simulink model "MasterSubsystems"  (R2021b)
settings: Solver=FixedStepDiscrete  StartTime=0.0  StopTime=10.0  FixedStep=0.001  RelTol=1e-3
undefined symbols (not defined in the file): DiscIntNeverNeededParam
libraries: slpidlib x2
settings Model: TunableVars=dt,k1  TunableVarsStorageClass=Auto,Auto  TunableVarsTypeQualifier=,  Creator=rrai-HIL  LastModifiedBy=rrai-HIL
settings ConfigComp: PLC_TargetIDE=plcopen  PLC_MultiTBSigbuilderTimeRange=off  PLC_ReuseMLFcnVariable=on  PLC_InlineEnumCastFunction=off

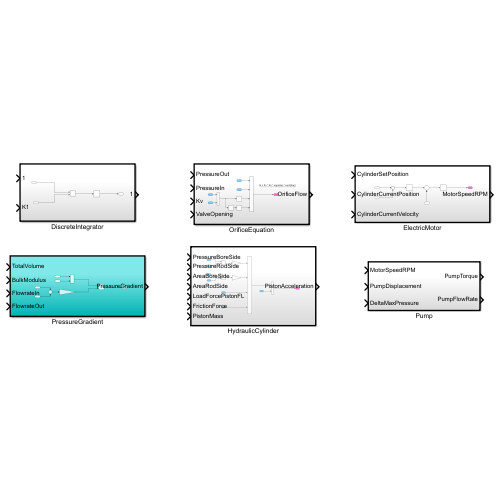
[thumbnail: Simulink's stored preview of the top-level diagram]
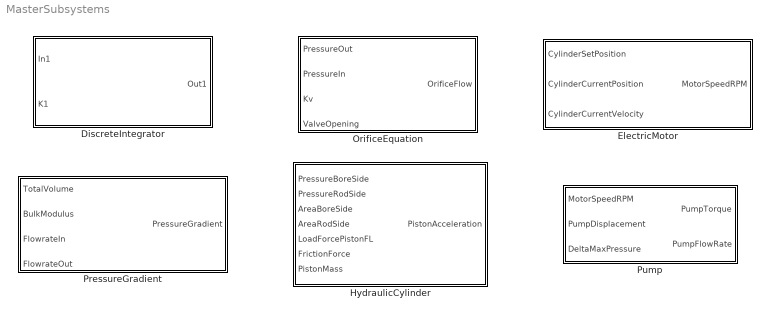
== system MasterSubsystems ==
  DiscreteIntegrator : Subsystem  TreatAsAtomicUnit=on
  ElectricMotor : Subsystem  TreatAsAtomicUnit=on
  HydraulicCylinder : Subsystem  TreatAsAtomicUnit=on
  OrificeEquation : Subsystem  TreatAsAtomicUnit=on
  PressureGradient : Subsystem  TreatAsAtomicUnit=on
  Pump : Subsystem  TreatAsAtomicUnit=on

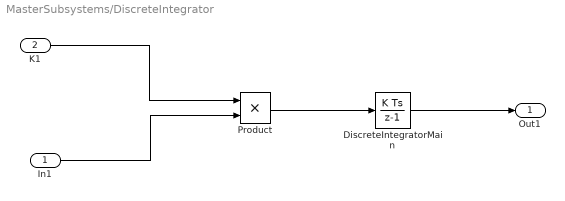
== system MasterSubsystems/DiscreteIntegrator ==
  In1 : Inport  OutDataTypeStr=single
  K1 : Inport  Port=2  OutDataTypeStr=single
  DiscreteIntegratorMain : DiscreteIntegrator  SampleTime=-1  ICPrevOutput=DiscIntNeverNeededParam  ICPrevScaledInput=DiscIntNeverNeededParam
  Product : Product
  Out1 : Outport  OutDataTypeStr=single
  wires:
  DiscreteIntegratorMain/1 -> Out1/1
  In1/1 -> Product/2
  Product/1 -> DiscreteIntegratorMain/1
  K1/1 -> Product/1

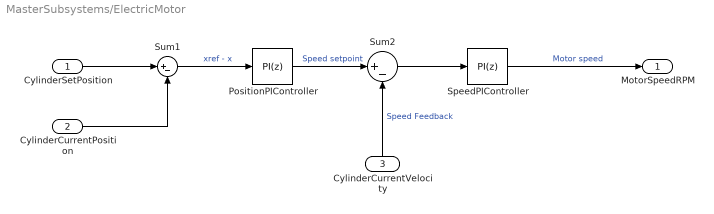
== system MasterSubsystems/ElectricMotor ==
  CylinderSetPosition : Inport
  CylinderCurrentPosition : Inport  Port=2
  CylinderCurrentVelocity : Inport  Port=3
  PositionPIController : slpidlib/PID Controller  Controller=PI  Form=Parallel  TimeDomain=Discrete-time  UseExternalTs=off  SampleTime=-1  IntegratorMethod=Forward Euler  FilterMethod=Forward Euler  ControllerParametersSource=internal  P=5  I=0.001  D=0  UseFilter=on  N=100  TunerSelectOption=Transfer Function Based (PID Tuner App)  InitialConditionSource=internal  InitialConditionForIntegrator=0  InitialConditionForFilter=0  DifferentiatorICPrevScaledInput=0  ExternalReset=none  TrackingMode=off  Kt=1  LimitOutput=on  SatLimitsSource=internal  UpperSaturationLimit=0.23  LowerSaturationLimit=-0.23  LinearizeAsGain=on  AntiWindupMode=none  Kb=1  POutMin=[]  POutMax=[]  IOutMin=[]  IOutMax=[]  DOutMin=[]  DOutMax=[]  NOutMin=[]  NOutMax=[]  SumOutMin=[]  SumOutMax=[]  SaturationOutMin=[]  SaturationOutMax=[]  PParamMin=[]  PParamMax=[]  IParamMin=[]  IParamMax=[]  DParamMin=[]  DParamMax=[]  NParamMin=[]  NParamMax=[]  KbParamMin=[]  KbParamMax=[]  KtParamMin=[]  KtParamMax=[]  KbOutMin=[]  KbOutMax=[]  KtOutMin=[]  KtOutMax=[]  IntegratorOutMin=[]  IntegratorOutMax=[]  FilterOutMin=[]  FilterOutMax=[]  SumI1OutMin=[]  SumI1OutMax=[]  SumI2OutMin=[]  SumI2OutMax=[]  SumI3OutMin=[]  SumI3OutMax=[]  SumI4OutMin=[]  SumI4OutMax=[]  SumDOutMin=[]  SumDOutMax=[]  DifferentiatorOutMin=[]  DifferentiatorOutMax=[]  FilterDiffOutCoefMin=[]  FilterDiffOutCoefMax=[]  ReciprocalOutMin=[]  ReciprocalOutMax=[]  SumDenOutMin=[]  SumDenOutMax=[]  SumNumOutMin=[]  SumNumOutMax=[]  DivideOutMin=[]  DivideOutMax=[]  UdiffTsProdOutMin=[]  UdiffTsProdOutMax=[]  NTsProdOutMin=[]  NTsProdOutMax=[]  UintegralTsProdOutMin=[]  UintegralTsProdOutMax=[]  UngainTsProdOutMin=[]  UngainTsProdOutMax=[]  IntegratorContinuousStateAttributes=''  IntegratorStateMustResolveToSignalObject=off  IntegratorRTWStateStorageClass=Auto  FilterContinuousStateAttributes=''  FilterStateMustResolveToSignalObject=off  FilterRTWStateStorageClass=Auto  ParallelPVariant=InternalParameters  IdealPVariant=Disabled  IVariant=InternalParameters  DVariant=Disabled  IntegratorVariant=Discrete  SatVariant=Enabled  AWVariant=Passthrough  PCopyVariant=Disabled  TRVariant=Disabled  FdbkBlocksVariant=Forward  IdealPFdbkVariant=Disabled  SatFdbkVariant=Disabled  DerivativeFilterVariant=Disabled  NVariant=Disabled  NCopyVariant=Disabled_SignalSpec  FilterICVariant=Disabled  IntegratorICVariant=InternalICs  ExternalResetVariant=Disabled  TRSumVariant=Passthrough  SumFdbkVariant=Disabled  SumVariant=Sum_PI  TsampFilterVariant=InternalTs  TsampNgainVariant=Passthrough  TsampIntegralVariant=Passthrough  ExternalSaturationOutDataTypeStr=Inherit: Same as second input
  SpeedPIController : slpidlib/PID Controller  Controller=PI  Form=Parallel  TimeDomain=Discrete-time  UseExternalTs=off  SampleTime=-1  IntegratorMethod=Forward Euler  FilterMethod=Forward Euler  ControllerParametersSource=internal  P=2000  I=0.01  D=0  UseFilter=on  N=100  TunerSelectOption=Transfer Function Based (PID Tuner App)  InitialConditionSource=internal  InitialConditionForIntegrator=0  InitialConditionForFilter=0  DifferentiatorICPrevScaledInput=0  ExternalReset=none  TrackingMode=off  Kt=1  LimitOutput=off  SatLimitsSource=internal  UpperSaturationLimit=0.23  LowerSaturationLimit=-0.23  LinearizeAsGain=on  AntiWindupMode=none  Kb=1  POutMin=[]  POutMax=[]  IOutMin=[]  IOutMax=[]  DOutMin=[]  DOutMax=[]  NOutMin=[]  NOutMax=[]  SumOutMin=[]  SumOutMax=[]  SaturationOutMin=[]  SaturationOutMax=[]  PParamMin=[]  PParamMax=[]  IParamMin=[]  IParamMax=[]  DParamMin=[]  DParamMax=[]  NParamMin=[]  NParamMax=[]  KbParamMin=[]  KbParamMax=[]  KtParamMin=[]  KtParamMax=[]  KbOutMin=[]  KbOutMax=[]  KtOutMin=[]  KtOutMax=[]  IntegratorOutMin=[]  IntegratorOutMax=[]  FilterOutMin=[]  FilterOutMax=[]  SumI1OutMin=[]  SumI1OutMax=[]  SumI2OutMin=[]  SumI2OutMax=[]  SumI3OutMin=[]  SumI3OutMax=[]  SumI4OutMin=[]  SumI4OutMax=[]  SumDOutMin=[]  SumDOutMax=[]  DifferentiatorOutMin=[]  DifferentiatorOutMax=[]  FilterDiffOutCoefMin=[]  FilterDiffOutCoefMax=[]  ReciprocalOutMin=[]  ReciprocalOutMax=[]  SumDenOutMin=[]  SumDenOutMax=[]  SumNumOutMin=[]  SumNumOutMax=[]  DivideOutMin=[]  DivideOutMax=[]  UdiffTsProdOutMin=[]  UdiffTsProdOutMax=[]  NTsProdOutMin=[]  NTsProdOutMax=[]  UintegralTsProdOutMin=[]  UintegralTsProdOutMax=[]  UngainTsProdOutMin=[]  UngainTsProdOutMax=[]  IntegratorContinuousStateAttributes=''  IntegratorStateMustResolveToSignalObject=off  IntegratorRTWStateStorageClass=Auto  FilterContinuousStateAttributes=''  FilterStateMustResolveToSignalObject=off  FilterRTWStateStorageClass=Auto  ParallelPVariant=InternalParameters  IdealPVariant=Disabled  IVariant=InternalParameters  DVariant=Disabled  IntegratorVariant=Discrete  SatVariant=Disabled  AWVariant=Passthrough  PCopyVariant=Disabled  TRVariant=Disabled  FdbkBlocksVariant=Forward  IdealPFdbkVariant=Disabled  SatFdbkVariant=Disabled  DerivativeFilterVariant=Disabled  NVariant=Disabled  NCopyVariant=Disabled_SignalSpec  FilterICVariant=Disabled  IntegratorICVariant=InternalICs  ExternalResetVariant=Disabled  TRSumVariant=Passthrough  SumFdbkVariant=Disabled  SumVariant=Sum_PI  TsampFilterVariant=InternalTs  TsampNgainVariant=Passthrough  TsampIntegralVariant=Passthrough  ExternalSaturationOutDataTypeStr=Inherit: Same as second input
  Sum1 : Sum  Inputs=|+-
  Sum2 : Sum  Inputs=|+-
  MotorSpeedRPM : Outport
  wires:
  Sum2/1 -> SpeedPIController/1
  CylinderSetPosition/1 -> Sum1/1
  PositionPIController/1 -> Sum2/1  "Speed setpoint"
  SpeedPIController/1 -> MotorSpeedRPM/1  "Motor speed"
  Sum1/1 -> PositionPIController/1  "xref - x"
  CylinderCurrentPosition/1 -> Sum1/2
  CylinderCurrentVelocity/1 -> Sum2/2  "Speed Feedback"

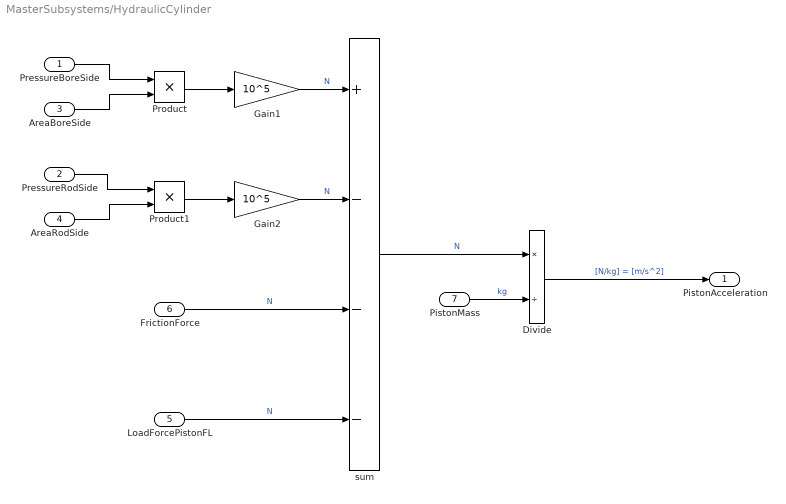
== system MasterSubsystems/HydraulicCylinder ==
  PressureBoreSide : Inport
  PressureRodSide : Inport  Port=2
  AreaBoreSide : Inport  Port=3
  AreaRodSide : Inport  Port=4
  LoadForcePistonFL : Inport  Port=5
  FrictionForce : Inport  Port=6
  PistonMass : Inport  Port=7
  "Divide " : Product  Inputs=*/
  Gain1 : Gain  Gain=10^5
  Gain2 : Gain  Gain=10^5
  Product : Product
  Product1 : Product
  sum : Sum  Inputs=+---
  PistonAcceleration : Outport
  wires:
  FrictionForce/1 -> sum/3  "N"
  AreaBoreSide/1 -> Product/2
  AreaRodSide/1 -> Product1/2
  PressureRodSide/1 -> Product1/1
  PressureBoreSide/1 -> Product/1
  PistonMass/1 -> "Divide "/2  "kg"
  sum/1 -> "Divide "/1  "N"
  LoadForcePistonFL/1 -> sum/4  "N"
  Product1/1 -> Gain2/1
  Gain2/1 -> sum/2  "N"
  Product/1 -> Gain1/1
  Gain1/1 -> sum/1  "N"
  "Divide "/1 -> PistonAcceleration/1  "[N/kg] = [m/s^2]"

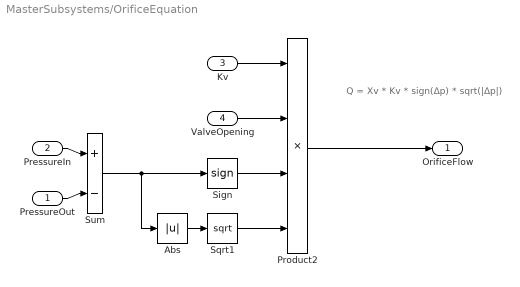
== system MasterSubsystems/OrificeEquation ==
  note: Q = Xv * Kv * sign(Δp) * sqrt(|Δp|)
  PressureOut : Inport
  PressureIn : Inport  Port=2
  Kv : Inport  Port=3
  ValveOpening : Inport  Port=4
  Abs : Abs
  Product2 : Product  Inputs=4
  Sign : Signum
  Sqrt1 : Sqrt  SaturateOnIntegerOverflow=on
  Sum : Sum  Inputs=+|-
  OrificeFlow : Outport
  wires:
  Kv/1 -> Product2/1
  Abs/1 -> Sqrt1/1
  PressureIn/1 -> Sum/1
  Sum/1 -> Abs/1, Sign/1
  PressureOut/1 -> Sum/2
  Product2/1 -> OrificeFlow/1
  ValveOpening/1 -> Product2/2
  Sqrt1/1 -> Product2/4
  Sign/1 -> Product2/3

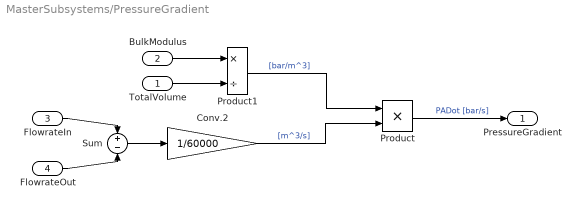
== system MasterSubsystems/PressureGradient ==
  TotalVolume : Inport
  BulkModulus : Inport  Port=2
  FlowrateIn : Inport  Port=3
  FlowrateOut : Inport  Port=4
  Conv.2 : Gain  Gain=1/60000
  Product : Product
  Product1 : Product  Inputs=*/
  Sum : Sum  Inputs=+-
  PressureGradient : Outport
  wires:
  Product1/1 -> Product/1  "[bar/m^3]"
  Product/1 -> PressureGradient/1  "PADot [bar/s]"
  Conv.2/1 -> Product/2  "[m^3/s]"
  BulkModulus/1 -> Product1/1
  TotalVolume/1 -> Product1/2
  Sum/1 -> Conv.2/1
  FlowrateOut/1 -> Sum/2
  FlowrateIn/1 -> Sum/1

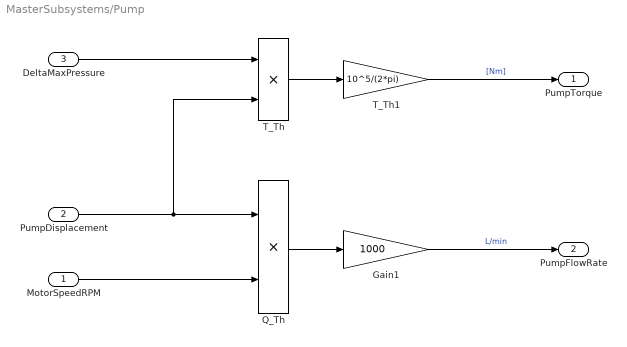
== system MasterSubsystems/Pump ==
  MotorSpeedRPM : Inport
  PumpDisplacement : Inport  Port=2
  DeltaMaxPressure : Inport  Port=3
  Gain1 : Gain  Gain=1000
  Q_Th : Product  RndMeth=Zero
  T_Th : Product  RndMeth=Zero
  T_Th1 : Gain  Gain=10^5/(2*pi)
  PumpTorque : Outport  VectorParamsAs1DForOutWhenUnconnected=off
  PumpFlowRate : Outport  Port=2  VectorParamsAs1DForOutWhenUnconnected=off
  wires:
  PumpDisplacement/1 -> T_Th/2, Q_Th/1
  Q_Th/1 -> Gain1/1
  T_Th/1 -> T_Th1/1
  T_Th1/1 -> PumpTorque/1  "[Nm]"
  MotorSpeedRPM/1 -> Q_Th/2
  Gain1/1 -> PumpFlowRate/1  "L/min"
  DeltaMaxPressure/1 -> T_Th/1
